simulink library "ddm"  (R2021b)
settings: Solver=VariableStepAuto  StartTime=0.0  StopTime=10.0  RelTol=1e-3
undefined symbols (not defined in the file or in its folder): ENUM_ADASACCSTA_ERROR, ENUM_ADASACCSTA_OFF, ENUM_ADASACCSTA_STANDBY, ENUM_ADASISASTA_OFF, ENUM_ALLOWMOV_ALLOWREADY, ENUM_APS, ENUM_BRKSTA_ERROR, ENUM_BRKSTA_OFF, ENUM_BRKSTA_ON, ENUM_BRKSW_INVALID, ENUM_BRKSW_OFF, ENUM_BRKSW_ON, ENUM_CHGPREACTERRSTA_OBCPRE, ENUM_DCDCFAULTSTA_ANYFAULTLV1, ENUM_DCDCFAULTSTA_ANYFAULTLV2, ENUM_DRIVETRAIN_AWD, ENUM_DRIVETRAIN_FWD, ENUM_DRIVETRAIN_RWD, ENUM_DRSEATSTA_INVALID, ENUM_EDUDRTSTA_NORMAL, ENUM_EPBSTA_APPLIED, ENUM_EPBSTA_RELEASED, ENUM_HVBATTREADYPRE_READY, ENUM_MCUWARN_LV0, ENUM_MCUWARN_LV1, ENUM_MCUWARN_LV2, ENUM_MCUWARN_LV3, ENUM_MCUWARN_NOERROR, ENUM_OBCFAULTSTA_ANYFAULT, ENUM_PAS_R2F2, ENUM_PDFAULT_BATTPDFAIL, ENUM_PDFAULT_DCDCDISABLE, ENUM_PDFAULT_MCUDISABLE, ENUM_PDFAULT_MCUDISCHRG, ENUM_POWERSTA_OFF, ENUM_POWERSTA_ON, ENUM_POWERSTA_READY, ENUM_POWERSTA_STANDBY, ENUM_PRESSINDI_LOW, ENUM_PUFAULT_BATTUPFAIL, ENUM_PUFAULT_DCDCENABLEFAIL, ENUM_PUFAULT_PRECHRGCHKFAIL, ENUM_PUFAULT_SAFETYCHKFAIL, ENUM_PUSTATE_COMPLETED, ENUM_PWRSTASW_OFF, ENUM_PWRSTASW_OFFA, ENUM_PWRSTASW_OFFCHVCHRG, ENUM_PWRSTASW_OFFCLVCHRG, ENUM_PWRSTASW_ON, ENUM_PWRSTASW_ONHVCHRG, ENUM_PWRSTASW_READY, ENUM_PWRSTASW_STANDBY, ENUM_RANGESTA_12IN, ENUM_SHIFTCOMMAND_D, ENUM_SHIFTCOMMAND_N, ENUM_SHIFTCOMMAND_P, ENUM_SHIFTCOMMAND_R, ENUM_VEHMALFUNLV_2ND, ENUM_VEHMALFUNLV_3RD, ENUM_VEHMALFUNLV_4TH ... (+835)
libraries: hcu_lib x750, $bdroot x12, simulink x5
(part 22 of 28)

== system ddm/DDM/DDM/PMM/power up and power down/MCU disable fail ==
  note: Diagnostics and Fault Handling
  note: Fail Safe Operation After Failure Decision
  note: Release Condition During Failure Detection
  note: Fail Safe Operation During Failure Detection
  note: Test Detection Criteria
  note: Release Condition After Failure Decision
  note: Test Pass Criteria
  task_time_s : Inport
  VPMM_PowerSta_enum : Inport  Port=2
  VPMM_PwrStaSW_enum : Inport  Port=3
  VPMM_PowerDownFault_enum : Inport  Port=4
  DTC_clear_request : Inport  Port=5
  Constant : Constant  Value=ENUM_PDFAULT_MCUDISABLE
  Constant10 : Constant  Value=KDDM_MCUDisDTC_cnt
  Constant11 : Constant  Value=KDDM_MCUDisPassSW_flg
  Constant15 : Constant  Value=KDDM_MCUDisCFSSW_flg
  Constant16 : Constant  Value=TRUE
  Constant17 : Constant  Value=KDDM_MCUDisPassTO_s
  Constant19 : Constant  Value=ENUM_POWERSTA_OFF
  Constant2 : Constant  Value=ENUM_PWRSTASW_OFF
  Constant20 : Constant  Value=KDDM_MCUDisDFSSW_flg
  Constant21 : Constant  Value=FALSE
  Constant22 : Constant  Value=ENUM_PWRSTASW_OFF
  Constant23 : Constant  Value=TRUE
  Constant24 : Constant  Value=TRUE
  Constant25 : Constant  Value=FALSE
  Constant27 : Constant  Value=FALSE
  Constant38 : Constant  Commented=on  Value=KDDM_MCUDisDetTO_s
  Constant40 : Constant  Commented=on  Value=KDDM_MCUDisDTC_cnt
  Constant43 : Constant  Value=KDDM_MCUDisPassTO_s
  Constant44 : Constant  Value=KDDM_MCUDisDetSW_flg
  DTC_Couter : hcu_lib/Basic_Blocks/DTC_Couter
  DTC_Info : hcu_lib/Basic_Blocks/DTC_Info
  Data Type Conversion1 : DataTypeConversion  OutDataTypeStr=uint8
  Equal1 : RelationalOperator  Operator===  OutDataTypeStr=boolean  RndMeth=Simplest
  Equal2 : RelationalOperator  Operator=~=  OutDataTypeStr=boolean  RndMeth=Simplest
  Equal4 : RelationalOperator  Operator=~=  OutDataTypeStr=boolean  RndMeth=Simplest
  Equal6 : RelationalOperator  OutDataTypeStr=boolean  RndMeth=Simplest
  Equal7 : RelationalOperator  Operator===  OutDataTypeStr=boolean  RndMeth=Simplest
  From48 : From  Commented=on  GotoTag=task_time_s
  Goto24 : Goto  Commented=on  GotoTag=VDDM_EDriveSysErrVCUErr_flg
  Logical Operator1 : Logic  Operator=NOT  AllPortsSameDT=off  OutDataTypeStr=boolean
  Logical Operator12 : Logic  AllPortsSameDT=off  OutDataTypeStr=boolean
  Logical Operator15 : Logic  AllPortsSameDT=off  OutDataTypeStr=boolean
  Logical Operator18 : Logic  AllPortsSameDT=off  OutDataTypeStr=boolean
  Logical Operator19 : Logic  Inputs=3  AllPortsSameDT=off  OutDataTypeStr=boolean
  Logical Operator2 : Logic  Operator=OR  AllPortsSameDT=off  OutDataTypeStr=boolean
  Logical Operator3 : Logic  Operator=OR  Inputs=3  AllPortsSameDT=off  OutDataTypeStr=boolean
  Logical Operator4 : Logic  Operator=OR  AllPortsSameDT=off  OutDataTypeStr=boolean
  Logical Operator6 : Logic  Operator=NOT  AllPortsSameDT=off  OutDataTypeStr=boolean
  Logical Operator8 : Logic  Operator=OR  AllPortsSameDT=off  OutDataTypeStr=boolean
  Relay : Relay  OnSwitchValue=ONE_INT  OffSwitchValue=ZERO_INT
  SR_Latch1 : Subsystem  mask(SR_Latch){}
      mask help: SR latch function.
  SR_Latch3 : hcu_lib/Basic_Blocks/SR_Latch
  SR_Latch4 : hcu_lib/Basic_Blocks/SR_Latch
  Switch{,1,4..5} (4 alike) : Switch  Criteria=u2 ~= 0
  Test Detection Criteria : hcu_lib/Basic_Blocks/Test Detection Criteria  Commented=on
  Timer1 : hcu_lib/Basic_Blocks/Timer
  VDDM_MCUDisDTC_raw32 : Outport
  wires:
  [DTC_clear_request] -> Logical Operator3/3
  [VDDM_MCUDisCFS_flg] -> Logical Operator4/1
  Constant44/1 -> Logical Operator19/2
  [VDDM_MCUDisCFSRls_flg] -> Logical Operator2/1
  Logical Operator2/1 -> SR_Latch4/2
  Logical Operator1/1 -> Logical Operator19/3
  Constant10/1 -> DTC_Couter/3
  [VDDM_MCUDisDTC_cnt] -> Relay/1
  Logical Operator4/1 -> SR_Latch3/2
  Logical Operator12/1 -> [VDDM_MCUDisDFS_flg]  "VDDM_MCUDisDFS_flg"
  Constant20/1 -> Logical Operator12/1
  SR_Latch3/1 -> Logical Operator12/2
  Relay/1 -> SR_Latch3/1
  [DTC_clear_request] -> Logical Operator2/2
  [VDDM_MCUDisDet_flg] -> Logical Operator19/1
  Logical Operator3/1 -> Logical Operator15/1
  Logical Operator18/1 -> [VDDM_MCUDisCFS_flg]  "VDDM_MCUDisCFS_flg"
  Data Type Conversion1/1 -> [VDDM_MCUDisDTC_cnt]  "VDDM_MCUDisDTC_cnt"
  Constant15/1 -> Logical Operator18/2
  Constant11/1 -> Logical Operator15/2
  [DTC_clear_request] -> Logical Operator4/2
  [VDDM_MCUDisPass_flg] -> Logical Operator3/1
  [DTC_clear_request] -> Logical Operator1/1
  Logical Operator15/1 -> DTC_Couter/2
  DTC_Couter/1 -> SR_Latch4/1
  DTC_Couter/2 -> Data Type Conversion1/1
  [VDDM_MCUDisCFSRls_flg] -> Logical Operator3/2
  SR_Latch4/1 -> Logical Operator18/1
  Logical Operator19/1 -> DTC_Couter/1
  [DTC_clear_request] -> DTC_Info/4
  Constant38/1 -> Test Detection Criteria/4
  [VDDM_MCUDisDet_flg] -> DTC_Info/1
  [VDDM_MCUDisCFS_flg] -> DTC_Info/3
  [VDDM_MCUDisPass_flg] -> DTC_Info/2
  DTC_Info/1 -> VDDM_MCUDisDTC_raw32/1  "VDDM_MCUDisDTC_raw32"
  Equal1/1 -> [VDDM_MCUDisChk_flg]
  Constant2/1 -> Equal2/2
  [VPMM_PwrStaSW_enum] -> Equal2/1
  DTC_clear_request/1 -> [DTC_clear_request]
  VPMM_PowerDownFault_enum/1 -> Equal1/1
  Constant/1 -> Equal1/2
  Timer1/1 -> Equal6/1
  [task_time_s] -> Timer1/3
  Constant40/1 -> Test Detection Criteria/3
  [DTC_clear_request] -> Logical Operator8/2
  Constant22/1 -> Equal4/2
  SR_Latch1/1(latched) -> [VDDM_MCUDisPass_flg]  "VDDM_MCUDisPass_flg"
  Logical Operator6/1 -> Timer1/1
  Switch5/1 -> [VDDM_MCUDisDet_flg]  "VDDM_MCUDisDet_flg"
  Constant24/1 -> Switch4/1
  Logical Operator8/1 -> Switch4/2
  Equal7/1 -> Logical Operator8/1
  From48/1 -> Test Detection Criteria/2
  Switch/1 -> Goto24/1
  Constant21/1 -> Switch/3
  Equal6/1 -> SR_Latch1/1(set)
  Constant19/1 -> Equal7/2
  Switch4/1 -> [VDDM_MCUDisCFSRls_flg]  "VDDM_MCUDisCFSRls_flg"
  [VDDM_MCUDisCFS_flg] -> Switch/2
  [VDDM_MCUDisChk_flg] -> Switch5/1
  Constant16/1 -> Switch/1
  Constant25/1 -> Switch4/3
  Constant27/1 -> Switch5/3
  Constant43/1 -> Timer1/4
  Constant17/1 -> Equal6/2
  [VPMM_PwrStaSW_enum] -> Equal4/1
  [VPMM_PowerSta_enum] -> Equal7/1
  Switch1/1 -> Timer1/2, SR_Latch1/2(reset), Logical Operator6/1
  Equal4/1 -> Switch5/2
  Equal2/1 -> Switch1/2
  [VDDM_MCUDisChk_flg] -> Switch1/1
  Constant23/1 -> Switch1/3
  VPMM_PowerSta_enum/1 -> [VPMM_PowerSta_enum]
  VPMM_PwrStaSW_enum/1 -> [VPMM_PwrStaSW_enum]
  task_time_s/1 -> [task_time_s]

== system ddm/DDM/DDM/PMM/power up and power down/MCU ready for precharge fail ==
  note: Diagnostics and Fault Handling
  note: Fail Safe Operation After Failure Decision
  note: Release Condition After Failure Decision
  note: Release Condition During Failure Detection
  note: Test Detection Criteria
  note: Fail Safe Operation During Failure Detection
  note: Test Pass Criteria
  task_time_s : Inport
  VPMM_PowerSta_enum : Inport  Port=2
  VPMM_PwrStaSW_enum : Inport  Port=3
  VPMM_MCUReady4Pre_flg : Inport  Port=4
  VPMM_PowerUpFault_enum : Inport  Port=5
  DTC_clear_request : Inport  Port=6
  VPMM_PowerUpState_enum : Inport  Port=7
  Constant : Constant  Value=ENUM_PUFAULT_PRECHRGCHKFAIL
  Constant1 : Constant  Value=ENUM_PUSTATE_COMPLETED
  Constant10 : Constant  Value=KDDM_MCU4PreDTC_cnt
  Constant11 : Constant  Value=KDDM_MCU4PrePassSW_flg
  Constant15 : Constant  Value=KDDM_MCU4PreCFSSW_flg
  Constant16 : Constant  Value=TRUE
  Constant19 : Constant  Value=ENUM_POWERSTA_OFF
  Constant{2,21,25,27} (4 alike) : Constant  Value=FALSE
  Constant20 : Constant  Value=KDDM_MCU4PreDFSSW_flg
  Constant23 : Constant  Value=TRUE
  Constant24 : Constant  Value=TRUE
  Constant26 : Constant  Value=ENUM_PWRSTASW_OFF
  Constant38 : Constant  Commented=on  Value=KDDM_MCU4PreDetTO_s
  Constant40 : Constant  Commented=on  Value=KDDM_MCU4PreDTC_cnt
  Constant43 : Constant  Value=KDDM_MCU4PrePassTO_s
  Constant44 : Constant  Value=KDDM_MCU4PreDetSW_flg
  Constant8 : Constant  Value=KDDM_MCU4PrePassTO_s
  DTC_Couter : hcu_lib/Basic_Blocks/DTC_Couter
  DTC_Info : hcu_lib/Basic_Blocks/DTC_Info
  Data Type Conversion1 : DataTypeConversion  OutDataTypeStr=uint8
  Equal : RelationalOperator  Operator=~=  OutDataTypeStr=boolean  RndMeth=Simplest
  Equal1 : RelationalOperator  Operator===  OutDataTypeStr=boolean  RndMeth=Simplest
  Equal2 : RelationalOperator  Operator===  OutDataTypeStr=boolean  RndMeth=Simplest
  Equal5 : RelationalOperator  OutDataTypeStr=boolean  RndMeth=Simplest
  Equal6 : RelationalOperator  Operator===  OutDataTypeStr=boolean  RndMeth=Simplest
  From48 : From  Commented=on  GotoTag=task_time_s
  Goto24 : Goto  Commented=on  GotoTag=VDDM_EDriveSysErrVCUErr_flg
  Logical Operator1 : Logic  Operator=OR  AllPortsSameDT=off  OutDataTypeStr=boolean
  Logical Operator{4,12,15,18} (4 alike) : Logic  AllPortsSameDT=off  OutDataTypeStr=boolean
  Logical Operator19 : Logic  Inputs=3  AllPortsSameDT=off  OutDataTypeStr=boolean
  Logical Operator2 : Logic  Operator=NOT  AllPortsSameDT=off  OutDataTypeStr=boolean
  Logical Operator3 : Logic  Operator=OR  Inputs=3  AllPortsSameDT=off  OutDataTypeStr=boolean
  Logical Operator5 : Logic  Operator=NOT  AllPortsSameDT=off  OutDataTypeStr=boolean
  Logical Operator6 : Logic  Operator=NOT  AllPortsSameDT=off  OutDataTypeStr=boolean
  Logical Operator7 : Logic  Operator=OR  AllPortsSameDT=off  OutDataTypeStr=boolean
  Logical Operator8 : Logic  Operator=OR  AllPortsSameDT=off  OutDataTypeStr=boolean
  Relay : Relay  OnSwitchValue=ONE_INT  OffSwitchValue=ZERO_INT
  SR_Latch1 : Subsystem  mask(SR_Latch){}
      mask help: SR latch function.
  SR_Latch3 : hcu_lib/Basic_Blocks/SR_Latch
  SR_Latch4 : hcu_lib/Basic_Blocks/SR_Latch
  Switch{,2,4..5} (4 alike) : Switch  Criteria=u2 ~= 0
  Test Detection Criteria : hcu_lib/Basic_Blocks/Test Detection Criteria  Commented=on
  Timer1 : hcu_lib/Basic_Blocks/Timer
  VDDM_MCU4PreDTC_raw32 : Outport
  wires:
  Constant15/1 -> Logical Operator18/2
  DTC_Couter/2 -> Data Type Conversion1/1
  [VDDM_MCU4PreCFS_flg] -> Logical Operator7/1
  [DTC_clear_request] -> Logical Operator7/2
  [VDDM_MCU4PreCFSRls_flg] -> Logical Operator1/1
  Constant10/1 -> DTC_Couter/3
  Logical Operator12/1 -> [VDDM_MCU4PreDFS_flg]  "VDDM_MCU4PreDFS_flg"
  [VDDM_MCU4PreDTC_cnt] -> Relay/1
  Constant44/1 -> Logical Operator19/2
  DTC_Couter/1 -> SR_Latch4/1
  Constant11/1 -> Logical Operator15/2
  SR_Latch4/1 -> Logical Operator18/1
  [VDDM_MCU4PreDet_flg] -> Logical Operator19/1
  Constant20/1 -> Logical Operator12/1
  Relay/1 -> SR_Latch3/1
  Data Type Conversion1/1 -> [VDDM_MCU4PreDTC_cnt]  "VDDM_MCU4PreDTC_cnt"
  Logical Operator15/1 -> DTC_Couter/2
  Logical Operator18/1 -> [VDDM_MCU4PreCFS_flg]  "VDDM_MCU4PreCFS_flg"
  Logical Operator19/1 -> DTC_Couter/1
  Logical Operator7/1 -> SR_Latch3/2
  [DTC_clear_request] -> Logical Operator3/3
  [DTC_clear_request] -> Logical Operator2/1
  Logical Operator3/1 -> Logical Operator15/1
  Logical Operator1/1 -> SR_Latch4/2
  [VDDM_MCU4PrePass_flg] -> Logical Operator3/1
  [VDDM_MCU4PreCFSRls_flg] -> Logical Operator3/2
  [DTC_clear_request] -> Logical Operator1/2
  Logical Operator2/1 -> Logical Operator19/3
  SR_Latch3/1 -> Logical Operator12/2
  [VPMM_PowerUpState_enum] -> Equal2/1
  Constant1/1 -> Equal2/2
  Constant2/1 -> Switch2/1
  VPMM_PowerUpState_enum/1 -> [VPMM_PowerUpState_enum]
  [DTC_clear_request] -> DTC_Info/4
  Constant38/1 -> Test Detection Criteria/4
  [VDDM_MCU4PreDet_flg] -> DTC_Info/1
  [VDDM_MCU4PreCFS_flg] -> DTC_Info/3
  DTC_Info/1 -> VDDM_MCU4PreDTC_raw32/1  "VDDM_MCU4PreDTC_raw32"
  [VDDM_MCU4PrePass_flg] -> DTC_Info/2
  VPMM_MCUReady4Pre_flg/1 -> Logical Operator5/1
  Logical Operator4/1 -> [VDDM_MCU4PreChk_flg]
  Equal1/1 -> Logical Operator4/2
  Logical Operator5/1 -> Logical Operator4/1
  VPMM_PowerUpFault_enum/1 -> Equal1/1
  Constant/1 -> Equal1/2
  DTC_clear_request/1 -> [DTC_clear_request]
  Switch2/1 -> Logical Operator6/1, Timer1/2, SR_Latch1/2(reset)
  Timer1/1 -> Equal5/1
  [VDDM_MCU4PreChk_flg] -> Switch5/1
  SR_Latch1/1(latched) -> [VDDM_MCU4PrePass_flg]  "VDDM_MCU4PrePass_flg"
  Equal6/1 -> Logical Operator8/1
  Constant23/1 -> Switch2/3
  Constant19/1 -> Equal6/2
  Logical Operator6/1 -> Timer1/1
  Constant27/1 -> Switch5/3
  Logical Operator8/1 -> Switch4/2
  Equal/1 -> Switch5/2
  [VDDM_MCU4PreCFS_flg] -> Switch/2
  [DTC_clear_request] -> Logical Operator8/2
  Switch5/1 -> [VDDM_MCU4PreDet_flg]  "VDDM_MCU4PreDet_flg"
  [VPMM_PwrStaSW_enum] -> Equal/1
  Constant43/1 -> Timer1/4
  Constant40/1 -> Test Detection Criteria/3
  Constant24/1 -> Switch4/1
  Constant8/1 -> Equal5/2
  Constant25/1 -> Switch4/3
  Constant21/1 -> Switch/3
  Equal5/1 -> SR_Latch1/1(set)
  Switch4/1 -> [VDDM_MCU4PreCFSRls_flg]  "VDDM_MCU4PreCFSRls_flg"
  Constant26/1 -> Equal/2
  Constant16/1 -> Switch/1
  Switch/1 -> Goto24/1
  [VPMM_PowerSta_enum] -> Equal6/1
  From48/1 -> Test Detection Criteria/2
  Equal2/1 -> Switch2/2
  [task_time_s] -> Timer1/3
  VPMM_PowerSta_enum/1 -> [VPMM_PowerSta_enum]
  VPMM_PwrStaSW_enum/1 -> [VPMM_PwrStaSW_enum]
  task_time_s/1 -> [task_time_s]

== system ddm/DDM/DDM/PMM/power up and power down/Mid level system safety check fail ==
  note: Diagnostics and Fault Handling
  note: Test Detection Criteria
  note: Release Condition After Failure Decision
  note: Fail Safe Operation After Failure Decision
  note: Fail Safe Operation During Failure Detection
  note: Release Condition During Failure Detection
  note: Test Pass Criteria
  task_time_s : Inport
  VPMM_PowerSta_enum : Inport  Port=2
  VPMM_PwrStaSW_enum : Inport  Port=3
  VDDM_MidLvSaChkChk_flg : Inport  Port=4
  VPMM_PowerUpFault_enum : Inport  Port=5
  DTC_clear_request : Inport  Port=6
  VPMM_PowerUpState_enum : Inport  Port=7
  Constant : Constant  Value=ENUM_PUFAULT_SAFETYCHKFAIL
  Constant1 : Constant  Value=ENUM_PUSTATE_COMPLETED
  Constant10 : Constant  Value=KDDM_MidLvSaChkDTC_cnt
  Constant11 : Constant  Value=KDDM_MidLvSaChkPassSW_flg
  Constant15 : Constant  Value=KDDM_MidLvSaChkCFSSW_flg
  Constant16 : Constant  Value=TRUE
  Constant19 : Constant  Value=ENUM_POWERSTA_OFF
  Constant{2,21,25,27} (4 alike) : Constant  Value=FALSE
  Constant20 : Constant  Value=KDDM_MidLvSaChkDFSSW_flg
  Constant23 : Constant  Value=TRUE
  Constant24 : Constant  Value=TRUE
  Constant26 : Constant  Value=ENUM_PWRSTASW_OFF
  Constant38 : Constant  Commented=on  Value=KDDM_MidLvSaChkDetTO_s
  Constant40 : Constant  Commented=on  Value=KDDM_MidLvSaChkDTC_cnt
  Constant43 : Constant  Value=KDDM_MidLvSaChkPassTO_s
  Constant44 : Constant  Value=KDDM_MidLvSaChkDetSW_flg
  Constant8 : Constant  Value=KDDM_MidLvSaChkPassTO_s
  DTC_Couter : hcu_lib/Basic_Blocks/DTC_Couter
  DTC_Info : hcu_lib/Basic_Blocks/DTC_Info
  Data Type Conversion1 : DataTypeConversion  OutDataTypeStr=uint8
  Equal : RelationalOperator  Operator=~=  OutDataTypeStr=boolean  RndMeth=Simplest
  Equal1 : RelationalOperator  Operator===  OutDataTypeStr=boolean  RndMeth=Simplest
  Equal2 : RelationalOperator  Operator===  OutDataTypeStr=boolean  RndMeth=Simplest
  Equal5 : RelationalOperator  OutDataTypeStr=boolean  RndMeth=Simplest
  Equal6 : RelationalOperator  Operator===  OutDataTypeStr=boolean  RndMeth=Simplest
  From48 : From  Commented=on  GotoTag=task_time_s
  Goto24 : Goto  Commented=on  GotoTag=VDDM_EDriveSysErrVCUErr_flg
  Logical Operator1 : Logic  Operator=NOT  AllPortsSameDT=off  OutDataTypeStr=boolean
  Logical Operator{5,12,15,18} (4 alike) : Logic  AllPortsSameDT=off  OutDataTypeStr=boolean
  Logical Operator19 : Logic  Inputs=3  AllPortsSameDT=off  OutDataTypeStr=boolean
  Logical Operator2 : Logic  Operator=OR  AllPortsSameDT=off  OutDataTypeStr=boolean
  Logical Operator3 : Logic  Operator=OR  Inputs=3  AllPortsSameDT=off  OutDataTypeStr=boolean
  Logical Operator4 : Logic  Operator=NOT  AllPortsSameDT=off  OutDataTypeStr=boolean
  Logical Operator6 : Logic  Operator=NOT  AllPortsSameDT=off  OutDataTypeStr=boolean
  Logical Operator7 : Logic  Operator=OR  AllPortsSameDT=off  OutDataTypeStr=boolean
  Logical Operator8 : Logic  Operator=OR  AllPortsSameDT=off  OutDataTypeStr=boolean
  Relay : Relay  OnSwitchValue=ONE_INT  OffSwitchValue=ZERO_INT
  SR_Latch1 : Subsystem  mask(SR_Latch){}
      mask help: SR latch function.
  SR_Latch3 : hcu_lib/Basic_Blocks/SR_Latch
  SR_Latch4 : hcu_lib/Basic_Blocks/SR_Latch
  Switch{,2,4..5} (4 alike) : Switch  Criteria=u2 ~= 0
  Test Detection Criteria : hcu_lib/Basic_Blocks/Test Detection Criteria  Commented=on
  Timer1 : hcu_lib/Basic_Blocks/Timer
  VDDM_MidLvSaChkDTC_raw32 : Outport
  wires:
  Constant11/1 -> Logical Operator15/2
  Logical Operator18/1 -> [VDDM_MidLvSaChkCFS_flg]  "VDDM_MidLvSaChkCFS_flg"
  SR_Latch4/1 -> Logical Operator18/1
  [DTC_clear_request] -> Logical Operator2/2
  [DTC_clear_request] -> Logical Operator3/3
  [DTC_clear_request] -> Logical Operator7/2
  Logical Operator3/1 -> Logical Operator15/1
  Logical Operator2/1 -> SR_Latch4/2
  [VDDM_MidLvSaChkDet_flg] -> Logical Operator19/1
  Logical Operator1/1 -> Logical Operator19/3
  [DTC_clear_request] -> Logical Operator1/1
  [VDDM_MidLvSaChkCFSRls_flg] -> Logical Operator2/1
  Logical Operator7/1 -> SR_Latch3/2
  Relay/1 -> SR_Latch3/1
  DTC_Couter/2 -> Data Type Conversion1/1
  Logical Operator19/1 -> DTC_Couter/1
  [VDDM_MidLvSaChkDTC_cnt] -> Relay/1
  Logical Operator15/1 -> DTC_Couter/2
  [VDDM_MidLvSaChkPass_flg] -> Logical Operator3/1
  SR_Latch3/1 -> Logical Operator12/2
  Constant15/1 -> Logical Operator18/2
  Constant20/1 -> Logical Operator12/1
  [VDDM_MidLvSaChkCFS_flg] -> Logical Operator7/1
  DTC_Couter/1 -> SR_Latch4/1
  Data Type Conversion1/1 -> [VDDM_MidLvSaChkDTC_cnt]  "VDDM_MidLvSaChkDTC_cnt"
  Logical Operator12/1 -> [VDDM_MidLvSaChkDFS_flg]  "VDDM_MidLvSaChkDFS_flg"
  Constant44/1 -> Logical Operator19/2
  [VDDM_MidLvSaChkCFSRls_flg] -> Logical Operator3/2
  Constant10/1 -> DTC_Couter/3
  [VPMM_PowerUpState_enum] -> Equal2/1
  Constant1/1 -> Equal2/2
  Constant2/1 -> Switch2/1
  VPMM_PowerUpState_enum/1 -> [VPMM_PowerUpState_enum]
  [DTC_clear_request] -> DTC_Info/4
  Constant38/1 -> Test Detection Criteria/4
  [VDDM_MidLvSaChkDet_flg] -> DTC_Info/1
  [VDDM_MidLvSaChkCFS_flg] -> DTC_Info/3
  [VDDM_MidLvSaChkPass_flg] -> DTC_Info/2
  DTC_Info/1 -> VDDM_MidLvSaChkDTC_raw32/1  "VDDM_MidLvSaChkDTC_raw32"
  DTC_clear_request/1 -> [DTC_clear_request]
  VDDM_MidLvSaChkChk_flg/1 -> Logical Operator4/1
  Logical Operator5/1 -> [VDDM_MidLvSaChkChk_flg]
  VPMM_PowerUpFault_enum/1 -> Equal1/1
  Logical Operator4/1 -> Logical Operator5/1
  Equal1/1 -> Logical Operator5/2
  Constant/1 -> Equal1/2
  Timer1/1 -> Equal5/1
  [task_time_s] -> Timer1/3
  Constant40/1 -> Test Detection Criteria/3
  Switch2/1 -> SR_Latch1/2(reset), Timer1/2, Logical Operator6/1
  Logical Operator8/1 -> Switch4/2
  Constant27/1 -> Switch5/3
  Equal/1 -> Switch5/2
  [VPMM_PowerSta_enum] -> Equal6/1
  [DTC_clear_request] -> Logical Operator8/2
  Constant24/1 -> Switch4/1
  Constant43/1 -> Timer1/4
  Constant26/1 -> Equal/2
  SR_Latch1/1(latched) -> [VDDM_MidLvSaChkPass_flg]  "VDDM_MidLvSaChkPass_flg"
  Logical Operator6/1 -> Timer1/1
  Constant25/1 -> Switch4/3
  Switch5/1 -> [VDDM_MidLvSaChkDet_flg]  "VDDM_MidLvSaChkDet_flg"
  Switch/1 -> Goto24/1
  Constant23/1 -> Switch2/3
  From48/1 -> Test Detection Criteria/2
  Equal5/1 -> SR_Latch1/1(set)
  Equal6/1 -> Logical Operator8/1
  Equal2/1 -> Switch2/2
  [VDDM_MidLvSaChkCFS_flg] -> Switch/2
  Constant21/1 -> Switch/3
  Switch4/1 -> [VDDM_MidLvSaChkCFSRls_flg]  "VDDM_MidLvSaChkCFSRls_flg"
  [VPMM_PwrStaSW_enum] -> Equal/1
  Constant19/1 -> Equal6/2
  Constant8/1 -> Equal5/2
  [VDDM_MidLvSaChkChk_flg] -> Switch5/1
  Constant16/1 -> Switch/1
  task_time_s/1 -> [task_time_s]
  VPMM_PwrStaSW_enum/1 -> [VPMM_PwrStaSW_enum]
  VPMM_PowerSta_enum/1 -> [VPMM_PowerSta_enum]

== system ddm/DDM/DDM/PMM/power up and power down/OBC ready for precharge fail ==
  note: Diagnostics and Fault Handling
  note: Release Condition During Failure Detection
  note: Test Pass Criteria
  note: Test Detection Criteria
  note: Fail Safe Operation After Failure Decision
  note: Release Condition After Failure Decision
  note: Fail Safe Operation During Failure Detection
  task_time_s : Inport
  VPMM_PowerSta_enum : Inport  Port=2
  VPMM_PwrStaSW_enum : Inport  Port=3
  VPMM_HVChrgPreActionErrSta_enum : Inport  Port=4
  DTC_clear_request : Inport  Port=5
  Constant1 : Constant  Value=ENUM_PWRSTASW_OFFCLVCHRG
  Constant10 : Constant  Value=KDDM_OBC4PreDTC_cnt
  Constant11 : Constant  Value=KDDM_OBC4PrePassSW_flg
  Constant15 : Constant  Value=KDDM_OBC4PreCFSSW_flg
  Constant16 : Constant  Value=TRUE
  Constant17 : Constant  Value=KDDM_OBC4PrePassTO_s
  Constant18 : Constant  Value=ENUM_PWRSTASW_ONHVCHRG
  Constant19 : Constant  Value=ENUM_POWERSTA_OFF
  Constant2 : Constant  Value=ENUM_PWRSTASW_OFFCLVCHRG
  Constant20 : Constant  Value=KDDM_OBC4PreDFSSW_flg
  Constant{8,21,25,27} (4 alike) : Constant  Value=FALSE
  Constant23 : Constant  Value=TRUE
  Constant24 : Constant  Value=TRUE
  Constant26 : Constant  Value=ENUM_PWRSTASW_ON
  Constant3 : Constant  Value=ENUM_CHGPREACTERRSTA_OBCPRE
  Constant38 : Constant  Value=KDDM_OBC4PreDetTO_s
  Constant4 : Constant  Value=ENUM_PWRSTASW_ONHVCHRG
  Constant40 : Constant  Value=KDDM_OBC4PreDTC_cnt
  Constant43 : Constant  Value=KDDM_OBC4PrePassTO_s
  Constant44 : Constant  Value=KDDM_OBC4PreDetSW_flg
  Constant5 : Constant  Value=ENUM_PWRSTASW_ON
  Constant6 : Constant  Value=ENUM_PWRSTASW_OFFCHVCHRG
  Constant7 : Constant  Value=ENUM_PWRSTASW_OFFCHVCHRG
  DTC_Couter : hcu_lib/Basic_Blocks/DTC_Couter
  DTC_Info : hcu_lib/Basic_Blocks/DTC_Info
  Data Type Conversion1 : DataTypeConversion  OutDataTypeStr=uint8
  Equal{,1..4,6..9,24} (10 alike) : RelationalOperator  Operator===  OutDataTypeStr=boolean  RndMeth=Simplest
  Equal5 : RelationalOperator  OutDataTypeStr=boolean  RndMeth=Simplest
  Goto24 : Goto  Commented=on  GotoTag=VDDM_EDriveSysErrVCUErr_flg
  Logical Operator1 : Logic  Operator=OR  Inputs=4  AllPortsSameDT=off  OutDataTypeStr=boolean
  Logical Operator12 : Logic  AllPortsSameDT=off  OutDataTypeStr=boolean
  Logical Operator15 : Logic  AllPortsSameDT=off  OutDataTypeStr=boolean
  Logical Operator18 : Logic  AllPortsSameDT=off  OutDataTypeStr=boolean
  Logical Operator19 : Logic  Inputs=3  AllPortsSameDT=off  OutDataTypeStr=boolean
  Logical Operator2 : Logic  Operator=OR  Inputs=4  AllPortsSameDT=off  OutDataTypeStr=boolean
  Logical Operator3 : Logic  Operator=OR  Inputs=3  AllPortsSameDT=off  OutDataTypeStr=boolean
  Logical Operator4 : Logic  Operator=NOT  AllPortsSameDT=off  OutDataTypeStr=boolean
  Logical Operator5 : Logic  Operator=OR  AllPortsSameDT=off  OutDataTypeStr=boolean
  Logical Operator6 : Logic  Operator=NOT  AllPortsSameDT=off  OutDataTypeStr=boolean
  Logical Operator7 : Logic  Operator=OR  AllPortsSameDT=off  OutDataTypeStr=boolean
  Logical Operator8 : Logic  Operator=OR  AllPortsSameDT=off  OutDataTypeStr=boolean
  Relay : Relay  OnSwitchValue=ONE_INT  OffSwitchValue=ZERO_INT
  SR_Latch1 : Subsystem  mask(SR_Latch){}
      mask help: SR latch function.
  SR_Latch3 : hcu_lib/Basic_Blocks/SR_Latch
  SR_Latch4 : hcu_lib/Basic_Blocks/SR_Latch
  Switch{,1..2,4..5} (5 alike) : Switch  Criteria=u2 ~= 0
  Test Detection Criteria : hcu_lib/Basic_Blocks/Test Detection Criteria
  Timer1 : hcu_lib/Basic_Blocks/Timer
  VDDM_OBC4PreDTC_raw32 : Outport
  wires:
  Logical Operator12/1 -> [VDDM_OBC4PreDFS_flg]  "VDDM_OBC4PreDFS_flg"
  [DTC_clear_request] -> Logical Operator3/3
  Logical Operator4/1 -> Logical Operator19/3
  [DTC_clear_request] -> Logical Operator5/2
  Logical Operator7/1 -> SR_Latch3/2
  [VDDM_OBC4PreCFSRls_flg] -> Logical Operator5/1
  [VDDM_OBC4PreCFS_flg] -> Logical Operator7/1
  SR_Latch4/1 -> Logical Operator18/1
  Constant15/1 -> Logical Operator18/2
  Logical Operator3/1 -> Logical Operator15/1
  [VDDM_OBC4PrePass_flg] -> Logical Operator3/1
  Data Type Conversion1/1 -> [VDDM_OBC4PreDTC_cnt]  "VDDM_OBC4PreDTC_cnt"
  [DTC_clear_request] -> Logical Operator4/1
  [VDDM_OBC4PreDTC_cnt] -> Relay/1
  Constant20/1 -> Logical Operator12/1
  Constant11/1 -> Logical Operator15/2
  Constant44/1 -> Logical Operator19/2
  Logical Operator15/1 -> DTC_Couter/2
  [VDDM_OBC4PreCFSRls_flg] -> Logical Operator3/2
  Constant10/1 -> DTC_Couter/3
  [DTC_clear_request] -> Logical Operator7/2
  Logical Operator5/1 -> SR_Latch4/2
  Logical Operator18/1 -> [VDDM_OBC4PreCFS_flg]  "VDDM_OBC4PreCFS_flg"
  Logical Operator19/1 -> DTC_Couter/1
  DTC_Couter/2 -> Data Type Conversion1/1
  [VDDM_OBC4PreDet_flg] -> Logical Operator19/1
  DTC_Couter/1 -> SR_Latch4/1
  SR_Latch3/1 -> Logical Operator12/2
  Relay/1 -> SR_Latch3/1
  [VDDM_xxx_flg] -> SR_Latch1/2(reset)
  Switch2/1 -> Test Detection Criteria/1
  Constant8/1 -> Switch2/1
  [DTC_clear_request] -> Switch2/2
  Switch5/1 -> Switch2/3, [VDDM_xxx_flg]
  [DTC_clear_request] -> DTC_Info/4
  Constant38/1 -> Test Detection Criteria/4
  [VDDM_OBC4PreDet_flg] -> DTC_Info/1
  [VDDM_OBC4PreCFS_flg] -> DTC_Info/3
  [VDDM_OBC4PrePass_flg] -> DTC_Info/2
  DTC_Info/1 -> VDDM_OBC4PreDTC_raw32/1  "VDDM_OBC4PreDTC_raw32"
  [VPMM_PwrStaSW_enum] -> Equal9/1
  Constant4/1 -> Equal9/2
  Constant6/1 -> Equal7/2
  [VPMM_PwrStaSW_enum] -> Equal2/1
  Logical Operator1/1 -> Switch1/2
  Constant5/1 -> Equal2/2
  [VDDM_OBC4PreChk_flg] -> Switch1/1
  [VPMM_PwrStaSW_enum] -> Equal7/1
  Equal9/1 -> Logical Operator1/4
  Equal4/1 -> Logical Operator1/3
  Equal2/1 -> Logical Operator1/2
  Equal7/1 -> Logical Operator1/1
  [VPMM_PwrStaSW_enum] -> Equal4/1
  Constant2/1 -> Equal4/2
  Equal3/1 -> Logical Operator2/1
  Equal/1 -> Logical Operator2/2
  Equal1/1 -> Logical Operator2/3
  Equal8/1 -> Logical Operator2/4
  Constant1/1 -> Equal1/2
  [VPMM_PwrStaSW_enum] -> Equal1/1
  DTC_clear_request/1 -> [DTC_clear_request]
  [DTC_clear_request] -> Logical Operator8/2
  Constant23/1 -> Switch1/3
  Constant17/1 -> Equal5/2
  [VPMM_PwrStaSW_enum] -> Equal3/1
  [VPMM_PowerSta_enum] -> Equal6/1
  Constant27/1 -> Switch5/3
  Constant43/1 -> Timer1/4
  Logical Operator8/1 -> Switch4/2
  Constant25/1 -> Switch4/3
  Switch1/1 -> Timer1/2, Logical Operator6/1
  Constant16/1 -> Switch/1
  Constant26/1 -> Equal/2
  [VDDM_OBC4PreCFS_flg] -> Switch/2
  Constant19/1 -> Equal6/2
  Switch4/1 -> [VDDM_OBC4PreCFSRls_flg]  "VDDM_OBC4PreCFSRls_flg"
  [VDDM_OBC4PreChk_flg] -> Switch5/1
  Constant18/1 -> Equal8/2
  [VPMM_PwrStaSW_enum] -> Equal/1
  Constant21/1 -> Switch/3
  Equal5/1 -> SR_Latch1/1(set)
  Test Detection Criteria/1 -> [VDDM_OBC4PreDet_flg]  "VDDM_OBC4PreDet_flg"
  Logical Operator2/1 -> Switch5/2
  Equal6/1 -> Logical Operator8/1
  [task_time_s] -> Test Detection Criteria/2
  Switch/1 -> Goto24/1
  SR_Latch1/1(latched) -> [VDDM_OBC4PrePass_flg]  "VDDM_OBC4PrePass_flg"
  Logical Operator6/1 -> Timer1/1
  Constant24/1 -> Switch4/1
  Timer1/1 -> Equal5/1
  Constant7/1 -> Equal3/2
  Constant40/1 -> Test Detection Criteria/3
  [task_time_s] -> Timer1/3
  [VPMM_PwrStaSW_enum] -> Equal8/1
  Equal24/1 -> [VDDM_OBC4PreChk_flg]  "VDDM_OBC4PreChk_flg"
  VPMM_HVChrgPreActionErrSta_enum/1 -> Equal24/1
  Constant3/1 -> Equal24/2
  VPMM_PowerSta_enum/1 -> [VPMM_PowerSta_enum]
  VPMM_PwrStaSW_enum/1 -> [VPMM_PwrStaSW_enum]
  task_time_s/1 -> [task_time_s]

== system ddm/DDM/DDM/TPM/LFBatwarn/SR_Latch1 ==
  set : Inport
  reset : Inport  Port=2
  Logical Operator : Logic  AllPortsSameDT=off  OutDataTypeStr=boolean
  Logical Operator1 : Logic  Operator=NOT  AllPortsSameDT=off  OutDataTypeStr=boolean
  Switch1 : Switch  Criteria=u2 ~= 0  Threshold=0.5
      settings: AttributesFormatString=<Criteria=%<Criteria>>
  Switch2 : Switch  Criteria=u2 ~= 0  Threshold=0.5
      settings: AttributesFormatString=<Criteria=%<Criteria>>
  Unit Delay : UnitDelay  SampleTime=-1  HasFrameUpgradeWarning=on
  latched : Outport
  wires:
  Switch1/1 -> Unit Delay/1, latched/1
  set/1 -> Switch1/1, Logical Operator/1
  reset/1 -> Switch2/2, Logical Operator1/1
  Unit Delay/1 -> Switch2/3
  Switch2/1 -> Switch1/3
  Logical Operator/1 -> Switch1/2
  Logical Operator1/1 -> Logical Operator/2, Switch2/1

== system ddm/DDM/DDM/TPM/LFPressureLow/SR_Latch1 ==
  set : Inport
  reset : Inport  Port=2
  Logical Operator : Logic  AllPortsSameDT=off  OutDataTypeStr=boolean
  Logical Operator1 : Logic  Operator=NOT  AllPortsSameDT=off  OutDataTypeStr=boolean
  Switch1 : Switch  Criteria=u2 ~= 0  Threshold=0.5
      settings: AttributesFormatString=<Criteria=%<Criteria>>
  Switch2 : Switch  Criteria=u2 ~= 0  Threshold=0.5
      settings: AttributesFormatString=<Criteria=%<Criteria>>
  Unit Delay : UnitDelay  SampleTime=-1  HasFrameUpgradeWarning=on
  latched : Outport
  wires:
  Switch1/1 -> Unit Delay/1, latched/1
  set/1 -> Switch1/1, Logical Operator/1
  reset/1 -> Switch2/2, Logical Operator1/1
  Unit Delay/1 -> Switch2/3
  Switch2/1 -> Switch1/3
  Logical Operator/1 -> Switch1/2
  Logical Operator1/1 -> Logical Operator/2, Switch2/1

== system ddm/DDM/DDM/TPM/LFSensorfail/SR_Latch1 ==
  set : Inport
  reset : Inport  Port=2
  Logical Operator : Logic  AllPortsSameDT=off  OutDataTypeStr=boolean
  Logical Operator1 : Logic  Operator=NOT  AllPortsSameDT=off  OutDataTypeStr=boolean
  Switch1 : Switch  Criteria=u2 ~= 0  Threshold=0.5
      settings: AttributesFormatString=<Criteria=%<Criteria>>
  Switch2 : Switch  Criteria=u2 ~= 0  Threshold=0.5
      settings: AttributesFormatString=<Criteria=%<Criteria>>
  Unit Delay : UnitDelay  SampleTime=-1  HasFrameUpgradeWarning=on
  latched : Outport
  wires:
  Switch1/1 -> Unit Delay/1, latched/1
  set/1 -> Switch1/1, Logical Operator/1
  reset/1 -> Switch2/2, Logical Operator1/1
  Unit Delay/1 -> Switch2/3
  Switch2/1 -> Switch1/3
  Logical Operator/1 -> Switch1/2
  Logical Operator1/1 -> Logical Operator/2, Switch2/1

== system ddm/DDM/DDM/TPM/LFWheelTmpHigh/SR_Latch1 ==
  set : Inport
  reset : Inport  Port=2
  Logical Operator : Logic  AllPortsSameDT=off  OutDataTypeStr=boolean
  Logical Operator1 : Logic  Operator=NOT  AllPortsSameDT=off  OutDataTypeStr=boolean
  Switch1 : Switch  Criteria=u2 ~= 0  Threshold=0.5
      settings: AttributesFormatString=<Criteria=%<Criteria>>
  Switch2 : Switch  Criteria=u2 ~= 0  Threshold=0.5
      settings: AttributesFormatString=<Criteria=%<Criteria>>
  Unit Delay : UnitDelay  SampleTime=-1  HasFrameUpgradeWarning=on
  latched : Outport
  wires:
  Switch1/1 -> Unit Delay/1, latched/1
  set/1 -> Switch1/1, Logical Operator/1
  reset/1 -> Switch2/2, Logical Operator1/1
  Unit Delay/1 -> Switch2/3
  Switch2/1 -> Switch1/3
  Logical Operator/1 -> Switch1/2
  Logical Operator1/1 -> Logical Operator/2, Switch2/1

== system ddm/DDM/DDM/TPM/LRBatwarn/SR_Latch1 ==
  set : Inport
  reset : Inport  Port=2
  Logical Operator : Logic  AllPortsSameDT=off  OutDataTypeStr=boolean
  Logical Operator1 : Logic  Operator=NOT  AllPortsSameDT=off  OutDataTypeStr=boolean
  Switch1 : Switch  Criteria=u2 ~= 0  Threshold=0.5
      settings: AttributesFormatString=<Criteria=%<Criteria>>
  Switch2 : Switch  Criteria=u2 ~= 0  Threshold=0.5
      settings: AttributesFormatString=<Criteria=%<Criteria>>
  Unit Delay : UnitDelay  SampleTime=-1  HasFrameUpgradeWarning=on
  latched : Outport
  wires:
  Switch1/1 -> Unit Delay/1, latched/1
  set/1 -> Switch1/1, Logical Operator/1
  reset/1 -> Switch2/2, Logical Operator1/1
  Unit Delay/1 -> Switch2/3
  Switch2/1 -> Switch1/3
  Logical Operator/1 -> Switch1/2
  Logical Operator1/1 -> Logical Operator/2, Switch2/1

== system ddm/DDM/DDM/TPM/LRPressureLow/SR_Latch1 ==
  set : Inport
  reset : Inport  Port=2
  Logical Operator : Logic  AllPortsSameDT=off  OutDataTypeStr=boolean
  Logical Operator1 : Logic  Operator=NOT  AllPortsSameDT=off  OutDataTypeStr=boolean
  Switch1 : Switch  Criteria=u2 ~= 0  Threshold=0.5
      settings: AttributesFormatString=<Criteria=%<Criteria>>
  Switch2 : Switch  Criteria=u2 ~= 0  Threshold=0.5
      settings: AttributesFormatString=<Criteria=%<Criteria>>
  Unit Delay : UnitDelay  SampleTime=-1  HasFrameUpgradeWarning=on
  latched : Outport
  wires:
  Switch1/1 -> Unit Delay/1, latched/1
  set/1 -> Switch1/1, Logical Operator/1
  reset/1 -> Switch2/2, Logical Operator1/1
  Unit Delay/1 -> Switch2/3
  Switch2/1 -> Switch1/3
  Logical Operator/1 -> Switch1/2
  Logical Operator1/1 -> Logical Operator/2, Switch2/1

== system ddm/DDM/DDM/TPM/LRSensorfail/SR_Latch1 ==
  set : Inport
  reset : Inport  Port=2
  Logical Operator : Logic  AllPortsSameDT=off  OutDataTypeStr=boolean
  Logical Operator1 : Logic  Operator=NOT  AllPortsSameDT=off  OutDataTypeStr=boolean
  Switch1 : Switch  Criteria=u2 ~= 0  Threshold=0.5
      settings: AttributesFormatString=<Criteria=%<Criteria>>
  Switch2 : Switch  Criteria=u2 ~= 0  Threshold=0.5
      settings: AttributesFormatString=<Criteria=%<Criteria>>
  Unit Delay : UnitDelay  SampleTime=-1  HasFrameUpgradeWarning=on
  latched : Outport
  wires:
  Switch1/1 -> Unit Delay/1, latched/1
  set/1 -> Switch1/1, Logical Operator/1
  reset/1 -> Switch2/2, Logical Operator1/1
  Unit Delay/1 -> Switch2/3
  Switch2/1 -> Switch1/3
  Logical Operator/1 -> Switch1/2
  Logical Operator1/1 -> Logical Operator/2, Switch2/1

== system ddm/DDM/DDM/TPM/LRWheelTmpHigh/SR_Latch1 ==
  set : Inport
  reset : Inport  Port=2
  Logical Operator : Logic  AllPortsSameDT=off  OutDataTypeStr=boolean
  Logical Operator1 : Logic  Operator=NOT  AllPortsSameDT=off  OutDataTypeStr=boolean
  Switch1 : Switch  Criteria=u2 ~= 0  Threshold=0.5
      settings: AttributesFormatString=<Criteria=%<Criteria>>
  Switch2 : Switch  Criteria=u2 ~= 0  Threshold=0.5
      settings: AttributesFormatString=<Criteria=%<Criteria>>
  Unit Delay : UnitDelay  SampleTime=-1  HasFrameUpgradeWarning=on
  latched : Outport
  wires:
  Switch1/1 -> Unit Delay/1, latched/1
  set/1 -> Switch1/1, Logical Operator/1
  reset/1 -> Switch2/2, Logical Operator1/1
  Unit Delay/1 -> Switch2/3
  Switch2/1 -> Switch1/3
  Logical Operator/1 -> Switch1/2
  Logical Operator1/1 -> Logical Operator/2, Switch2/1

== system ddm/DDM/DDM/TPM/RFBatwarn/SR_Latch1 ==
  set : Inport
  reset : Inport  Port=2
  Logical Operator : Logic  AllPortsSameDT=off  OutDataTypeStr=boolean
  Logical Operator1 : Logic  Operator=NOT  AllPortsSameDT=off  OutDataTypeStr=boolean
  Switch1 : Switch  Criteria=u2 ~= 0  Threshold=0.5
      settings: AttributesFormatString=<Criteria=%<Criteria>>
  Switch2 : Switch  Criteria=u2 ~= 0  Threshold=0.5
      settings: AttributesFormatString=<Criteria=%<Criteria>>
  Unit Delay : UnitDelay  SampleTime=-1  HasFrameUpgradeWarning=on
  latched : Outport
  wires:
  Switch1/1 -> Unit Delay/1, latched/1
  set/1 -> Switch1/1, Logical Operator/1
  reset/1 -> Switch2/2, Logical Operator1/1
  Unit Delay/1 -> Switch2/3
  Switch2/1 -> Switch1/3
  Logical Operator/1 -> Switch1/2
  Logical Operator1/1 -> Logical Operator/2, Switch2/1

== system ddm/DDM/DDM/TPM/RFPressureLow/SR_Latch1 ==
  set : Inport
  reset : Inport  Port=2
  Logical Operator : Logic  AllPortsSameDT=off  OutDataTypeStr=boolean
  Logical Operator1 : Logic  Operator=NOT  AllPortsSameDT=off  OutDataTypeStr=boolean
  Switch1 : Switch  Criteria=u2 ~= 0  Threshold=0.5
      settings: AttributesFormatString=<Criteria=%<Criteria>>
  Switch2 : Switch  Criteria=u2 ~= 0  Threshold=0.5
      settings: AttributesFormatString=<Criteria=%<Criteria>>
  Unit Delay : UnitDelay  SampleTime=-1  HasFrameUpgradeWarning=on
  latched : Outport
  wires:
  Switch1/1 -> Unit Delay/1, latched/1
  set/1 -> Switch1/1, Logical Operator/1
  reset/1 -> Switch2/2, Logical Operator1/1
  Unit Delay/1 -> Switch2/3
  Switch2/1 -> Switch1/3
  Logical Operator/1 -> Switch1/2
  Logical Operator1/1 -> Logical Operator/2, Switch2/1

== system ddm/DDM/DDM/TPM/RFSensorfail/SR_Latch1 ==
  set : Inport
  reset : Inport  Port=2
  Logical Operator : Logic  AllPortsSameDT=off  OutDataTypeStr=boolean
  Logical Operator1 : Logic  Operator=NOT  AllPortsSameDT=off  OutDataTypeStr=boolean
  Switch1 : Switch  Criteria=u2 ~= 0  Threshold=0.5
      settings: AttributesFormatString=<Criteria=%<Criteria>>
  Switch2 : Switch  Criteria=u2 ~= 0  Threshold=0.5
      settings: AttributesFormatString=<Criteria=%<Criteria>>
  Unit Delay : UnitDelay  SampleTime=-1  HasFrameUpgradeWarning=on
  latched : Outport
  wires:
  Switch1/1 -> Unit Delay/1, latched/1
  set/1 -> Switch1/1, Logical Operator/1
  reset/1 -> Switch2/2, Logical Operator1/1
  Unit Delay/1 -> Switch2/3
  Switch2/1 -> Switch1/3
  Logical Operator/1 -> Switch1/2
  Logical Operator1/1 -> Logical Operator/2, Switch2/1

== system ddm/DDM/DDM/TPM/RFWheelTmpHigh/SR_Latch1 ==
  set : Inport
  reset : Inport  Port=2
  Logical Operator : Logic  AllPortsSameDT=off  OutDataTypeStr=boolean
  Logical Operator1 : Logic  Operator=NOT  AllPortsSameDT=off  OutDataTypeStr=boolean
  Switch1 : Switch  Criteria=u2 ~= 0  Threshold=0.5
      settings: AttributesFormatString=<Criteria=%<Criteria>>
  Switch2 : Switch  Criteria=u2 ~= 0  Threshold=0.5
      settings: AttributesFormatString=<Criteria=%<Criteria>>
  Unit Delay : UnitDelay  SampleTime=-1  HasFrameUpgradeWarning=on
  latched : Outport
  wires:
  Switch1/1 -> Unit Delay/1, latched/1
  set/1 -> Switch1/1, Logical Operator/1
  reset/1 -> Switch2/2, Logical Operator1/1
  Unit Delay/1 -> Switch2/3
  Switch2/1 -> Switch1/3
  Logical Operator/1 -> Switch1/2
  Logical Operator1/1 -> Logical Operator/2, Switch2/1

== system ddm/DDM/DDM/TPM/RRBatwarn/SR_Latch1 ==
  set : Inport
  reset : Inport  Port=2
  Logical Operator : Logic  AllPortsSameDT=off  OutDataTypeStr=boolean
  Logical Operator1 : Logic  Operator=NOT  AllPortsSameDT=off  OutDataTypeStr=boolean
  Switch1 : Switch  Criteria=u2 ~= 0  Threshold=0.5
      settings: AttributesFormatString=<Criteria=%<Criteria>>
  Switch2 : Switch  Criteria=u2 ~= 0  Threshold=0.5
      settings: AttributesFormatString=<Criteria=%<Criteria>>
  Unit Delay : UnitDelay  SampleTime=-1  HasFrameUpgradeWarning=on
  latched : Outport
  wires:
  Switch1/1 -> Unit Delay/1, latched/1
  set/1 -> Switch1/1, Logical Operator/1
  reset/1 -> Switch2/2, Logical Operator1/1
  Unit Delay/1 -> Switch2/3
  Switch2/1 -> Switch1/3
  Logical Operator/1 -> Switch1/2
  Logical Operator1/1 -> Logical Operator/2, Switch2/1

== system ddm/DDM/DDM/TPM/RRPressureLow/SR_Latch1 ==
  set : Inport
  reset : Inport  Port=2
  Logical Operator : Logic  AllPortsSameDT=off  OutDataTypeStr=boolean
  Logical Operator1 : Logic  Operator=NOT  AllPortsSameDT=off  OutDataTypeStr=boolean
  Switch1 : Switch  Criteria=u2 ~= 0  Threshold=0.5
      settings: AttributesFormatString=<Criteria=%<Criteria>>
  Switch2 : Switch  Criteria=u2 ~= 0  Threshold=0.5
      settings: AttributesFormatString=<Criteria=%<Criteria>>
  Unit Delay : UnitDelay  SampleTime=-1  HasFrameUpgradeWarning=on
  latched : Outport
  wires:
  Switch1/1 -> Unit Delay/1, latched/1
  set/1 -> Switch1/1, Logical Operator/1
  reset/1 -> Switch2/2, Logical Operator1/1
  Unit Delay/1 -> Switch2/3
  Switch2/1 -> Switch1/3
  Logical Operator/1 -> Switch1/2
  Logical Operator1/1 -> Logical Operator/2, Switch2/1

== system ddm/DDM/DDM/TPM/RRSensorfail/SR_Latch1 ==
  set : Inport
  reset : Inport  Port=2
  Logical Operator : Logic  AllPortsSameDT=off  OutDataTypeStr=boolean
  Logical Operator1 : Logic  Operator=NOT  AllPortsSameDT=off  OutDataTypeStr=boolean
  Switch1 : Switch  Criteria=u2 ~= 0  Threshold=0.5
      settings: AttributesFormatString=<Criteria=%<Criteria>>
  Switch2 : Switch  Criteria=u2 ~= 0  Threshold=0.5
      settings: AttributesFormatString=<Criteria=%<Criteria>>
  Unit Delay : UnitDelay  SampleTime=-1  HasFrameUpgradeWarning=on
  latched : Outport
  wires:
  Switch1/1 -> Unit Delay/1, latched/1
  set/1 -> Switch1/1, Logical Operator/1
  reset/1 -> Switch2/2, Logical Operator1/1
  Unit Delay/1 -> Switch2/3
  Switch2/1 -> Switch1/3
  Logical Operator/1 -> Switch1/2
  Logical Operator1/1 -> Logical Operator/2, Switch2/1

== system ddm/DDM/DDM/TPM/RRWheelTmpHigh/SR_Latch1 ==
  set : Inport
  reset : Inport  Port=2
  Logical Operator : Logic  AllPortsSameDT=off  OutDataTypeStr=boolean
  Logical Operator1 : Logic  Operator=NOT  AllPortsSameDT=off  OutDataTypeStr=boolean
  Switch1 : Switch  Criteria=u2 ~= 0  Threshold=0.5
      settings: AttributesFormatString=<Criteria=%<Criteria>>
  Switch2 : Switch  Criteria=u2 ~= 0  Threshold=0.5
      settings: AttributesFormatString=<Criteria=%<Criteria>>
  Unit Delay : UnitDelay  SampleTime=-1  HasFrameUpgradeWarning=on
  latched : Outport
  wires:
  Switch1/1 -> Unit Delay/1, latched/1
  set/1 -> Switch1/1, Logical Operator/1
  reset/1 -> Switch2/2, Logical Operator1/1
  Unit Delay/1 -> Switch2/3
  Switch2/1 -> Switch1/3
  Logical Operator/1 -> Switch1/2
  Logical Operator1/1 -> Logical Operator/2, Switch2/1
